simulink model "objectdetectandremember"  (R2023a)
settings: Solver=FixedStepDiscrete  StartTime=0.0  StopTime=200  FixedStep=0.01  RelTol=1e-3
undefined symbols (not defined in the file or in its folder): InputPWM, ticksPerRot, wheelR, WheelSpeed
libraries: mobileRoboticsTrainingLib x7, slpidlib x3
settings Model: Creator=Boitumelo  LastModifiedBy=Nate
settings DebuggingCC: UnconnectedInputMsg=warning  UnconnectedOutputMsg=warning  UnconnectedLineMsg=warning
settings ModelReferenceCC: EnableRefExpFcnMdlSchedulingChecks=on
settings RTWCC: DLArmComputeVersion=19.05

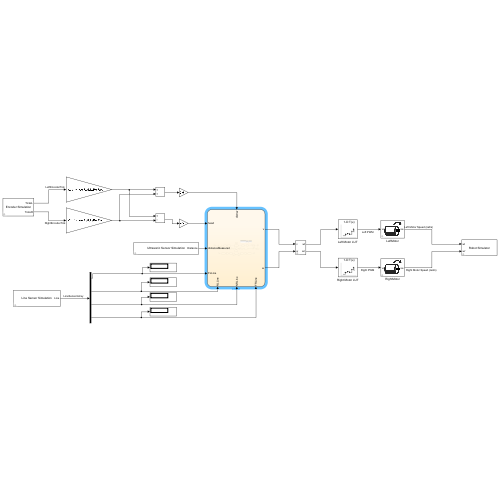
[thumbnail: Simulink's stored preview of the top-level diagram]
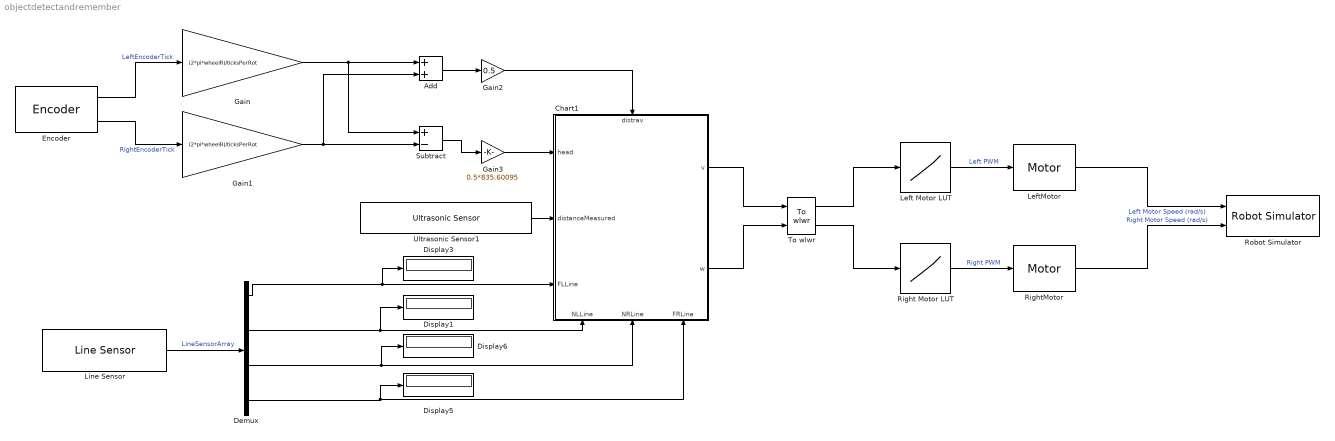
== system objectdetectandremember ==
  Add : Sum
  Chart1 : Stateflow chart  TreatAsAtomicUnit=on
      settings: PortSchema="{\"entries\":[{\"content\":{\"sides\":[{\"content\":{\"connectorIds\":[\"In6\",\"In5\",\"In7\"]},\"type\":\"ConnectorPlacement.EquallySpacedRectSide\",\"uuid\":\"27b5da46-073c-4681-8d78-c3525f10231c\"},{\"content\":{\"connectorIds\":[\"Out1\",\"Out2\"],\"side\":\"RIGHT\"},\"type\":\"ConnectorPlacement.EquallySpacedRectSide\",\"uuid\":\"84cbede5-d577-43ca-a2b5-5c732f2541a7\"},{\"content\":{\"connectorIds\":[\"In4\"],\"side\":\"TOP\"},\"type\":\"ConnectorPlacement.EquallySpacedRectSide\",\"uuid\":\"af8175f1-71d5-4094-87a9-6474fd0e0f31\"},{\"content\":{\"connectorIds\":[\"In1\",\"In2\",\"In3\"],\"side\":\"BOTTOM\"},\"type\":\"ConnectorPlacement.EquallySpacedRectSide\",\"uuid\":\"b4cb3a30-2878-490e-b77d-5d6435204590\"}]},\"type\":\"ConnectorPlacement.EquallySpacedConnector\",\"uuid\":\"b0958b58-2151-4ca2-a50e-e327f459f533\"}],\"packageUris\":[\"http://schema.mathworks.com/mf0/Connector/R2020b\"],\"version\":\"1.0\"}"
  Demux : Demux
  Display{1,3,5..6} (4 alike) : Display
  Encoder : mobileRoboticsTrainingLib/Encoder  axleLength=0.136  wheelR=0.031  ticksPerRot=20
      settings: SourceProductName=Mobile Robotics Training Library
  Gain : Gain  Gain=(2*pi*wheelR)/ticksPerRot
  Gain1 : Gain  Gain=(2*pi*wheelR)/ticksPerRot
  Gain2 : Gain  Gain=0.5
  Gain3 : Gain  Gain=0.5*835.60095
  Left Motor LUT : Lookup_n-D  NumberOfTableDimensions=1  BreakpointsForDimension1=WheelSpeed  Table=InputPWM  InterpMethod=Nearest  ExtrapMethod=Clip  InternalRulePriority=Speed  RndMeth=Simplest
  LeftMotor : mobileRoboticsTrainingLib/Motor  motorPlant=wheelMotorModel  sensorType=Speed
      settings: SourceProductName=Mobile Robotics Training Library
  Line Sensor : mobileRoboticsTrainingLib/Line Sensor  mapVariable=mapForSim  envVal=1000  lineVal=0  sensOff=[0.0643 0.0354; 0.0675 0.005; 0.0675 -0.005; 0.0643 -0.0354]
      settings: SourceProductName=Mobile Robotics Training Library
  Right Motor LUT : Lookup_n-D  NumberOfTableDimensions=1  BreakpointsForDimension1=WheelSpeed  Table=InputPWM  InterpMethod=Nearest  ExtrapMethod=Clip  InternalRulePriority=Speed  RndMeth=Simplest
  RightMotor : mobileRoboticsTrainingLib/Motor  motorPlant=wheelMotorModel  sensorType=Speed
      settings: SourceProductName=Mobile Robotics Training Library
  Robot Simulator : mobileRoboticsTrainingLib/Robot Simulator  Priority=99  mapVar=mapForSim  startX=1  startY=0.2  startTheta=90  axleLength=axleLength  wheelR=wheelR
      link override Wheel Radius: Value=0.031
      link override Wheel Spacing: Value=0.136
  Subtract : Sum  Inputs=+-
  To wlwr : mobileRoboticsTrainingLib/To wlwr  axleLength=axleLength  wheelR=wheelR
      link override change parameters: Gain=[1 +axleLength/2; 1 -axleLength/2]
  Ultrasonic Sensor1 : mobileRoboticsTrainingLib/Ultrasonic Sensor  mapVar=mapForSim  maxSenRange=2  minSenRange=0.02  senRes=0.01  sensOff=[0 0]
      link override Look up Distance Value/Subsystem/Look up Sensor Value/Lookup Obstacle Map/Direct Lookup Table (n-D): DiagnosticForOutOfRangeInput=Warning  TableIsInput=off
      settings: SourceProductName=Mobile Robotics Training Library
  wires:
  Right Motor LUT/1 -> RightMotor/1  "Right PWM"
  Left Motor LUT/1 -> LeftMotor/1  "Left PWM"
  To wlwr/1 -> Left Motor LUT/1
  To wlwr/2 -> Right Motor LUT/1
  RightMotor/1 -> Robot Simulator/2  "Right Motor Speed (rad/s)"
  LeftMotor/1 -> Robot Simulator/1  "Left Motor Speed (rad/s)"
  Line Sensor/1 -> Demux/1  "LineSensorArray"
  Demux/4 -> Display5/1, Chart1/3(FRLine)
  Demux/2 -> Display1/1, Chart1/1(NLLine)
  Demux/3 -> Display6/1, Chart1/2(NRLine)
  Chart1/2(w) -> To wlwr/2
  Chart1/1(v) -> To wlwr/1
  Ultrasonic Sensor1/1 -> Chart1/5(distanceMeasured)
  Gain2/1 -> Chart1/4(distrav)
  Encoder/1 -> Gain/1  "LeftEncoderTick"
  Gain/1 -> Subtract/1, Add/1
  Encoder/2 -> Gain1/1  "RightEncoderTick"
  Add/1 -> Gain2/1
  Demux/1 -> Display3/1, Chart1/7(FLLine)
  Gain1/1 -> Subtract/2, Add/2
  Gain3/1 -> Chart1/6(head)
  Subtract/1 -> Gain3/1

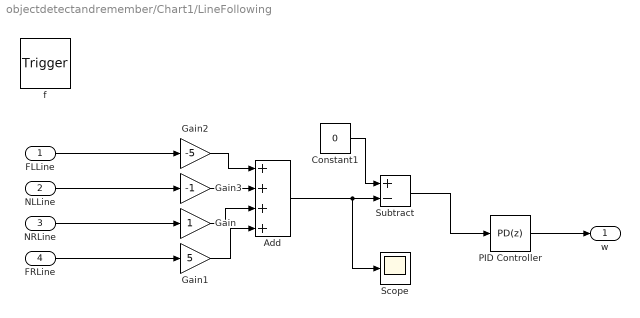
== system objectdetectandremember/Chart1/LineFollowing ==
  FLLine : Inport  OutDataTypeStr=double  PortDimensions=1
  NLLine : Inport  Port=2  OutDataTypeStr=double  PortDimensions=1
  NRLine : Inport  Port=3  OutDataTypeStr=double  PortDimensions=1
  FRLine : Inport  Port=4  OutDataTypeStr=double  PortDimensions=1
  f : TriggerPort  TriggerType=function-call  VariantControl=(inherit)
      settings: CopyFcn=Stateflow.SLINSF.SimulinkMan.removeBlockPreDeleteFcn  PreDeleteFcn=Stateflow.SLINSF.SimulinkMan.unsafePredeleteFcn
  Add : Sum  Inputs=++++
  Constant1 : Constant  Value=0
  Gain : Gain
  Gain1 : Gain  Gain=5
  Gain2 : Gain  Gain=-5
  Gain3 : Gain  Gain=-1
  PID Controller : slpidlib/PID Controller  Controller=PD  Form=Parallel  TimeDomain=Discrete-time  UseExternalTs=off  SampleTime=-1  IntegratorMethod=Forward Euler  FilterMethod=Forward Euler  ControllerParametersSource=internal  P=1  I=0  UseKiTs=off  D=1e-3  N=100  UseFilter=on  TunerSelectOption=Transfer Function Based (PID Tuner App)  InitialConditionSource=internal  InitialConditionForIntegrator=0  InitialConditionForFilter=0  DifferentiatorICPrevScaledInput=0  ExternalReset=none  TrackingMode=off  Kt=1  LimitOutput=off  SatLimitsSource=internal  UpperSaturationLimit=inf  LowerSaturationLimit=-inf  LinearizeAsGain=on  AntiWindupMode=none  Kb=1  LimitIntegrator=off  UpperIntegratorSaturationLimit=inf  LowerIntegratorSaturationLimit=-inf  POutMin=[]  POutMax=[]  IOutMin=[]  IOutMax=[]  DOutMin=[]  DOutMax=[]  NOutMin=[]  NOutMax=[]  SumOutMin=[]  SumOutMax=[]  SaturationOutMin=[]  SaturationOutMax=[]  PParamMin=[]  PParamMax=[]  IParamMin=[]  IParamMax=[]  DParamMin=[]  DParamMax=[]  NParamMin=[]  NParamMax=[]  KbParamMin=[]  KbParamMax=[]  KtParamMin=[]  KtParamMax=[]  KbOutMin=[]  KbOutMax=[]  KtOutMin=[]  KtOutMax=[]  IntegratorOutMin=[]  IntegratorOutMax=[]  FilterOutMin=[]  FilterOutMax=[]  SumI1OutMin=[]  SumI1OutMax=[]  SumI2OutMin=[]  SumI2OutMax=[]  SumI3OutMin=[]  SumI3OutMax=[]  SumI4OutMin=[]  SumI4OutMax=[]  SumDOutMin=[]  SumDOutMax=[]  DifferentiatorOutMin=[]  DifferentiatorOutMax=[]  FilterDiffOutCoefMin=[]  FilterDiffOutCoefMax=[]  ReciprocalOutMin=[]  ReciprocalOutMax=[]  SumDenOutMin=[]  SumDenOutMax=[]  SumNumOutMin=[]  SumNumOutMax=[]  DivideOutMin=[]  DivideOutMax=[]  UdiffTsProdOutMin=[]  UdiffTsProdOutMax=[]  NTsProdOutMin=[]  NTsProdOutMax=[]  UintegralTsProdOutMin=[]  UintegralTsProdOutMax=[]  UngainTsProdOutMin=[]  UngainTsProdOutMax=[]  ClampingZeroOutDataTypeStr=Inherit: Inherit via back propagation  ClampingZeroOutMin=[]  ClampingZeroOutMax=[]  FilterDenConstantOutDataTypeStr=Inherit: Inherit via back propagation  FilterDenConstantOutMin=[]  FilterDenConstantOutMax=[]  PCopyOutDataTypeStr=Inherit: Inherit via back propagation  PCopyOutMin=[]  PCopyOutMax=[]  NCopyOutDataTypeStr=Inherit: Inherit via back propagation  NCopyOutMin=[]  NCopyOutMax=[]  IntegratorContinuousStateAttributes=''  IntegratorStateMustResolveToSignalObject=off  IntegratorRTWStateStorageClass=Auto  FilterContinuousStateAttributes=''  FilterStateMustResolveToSignalObject=off  FilterRTWStateStorageClass=Auto  ParallelPVariant=InternalParameters  IdealPVariant=Disabled  IVariant=Disabled  DVariant=InternalParameters  IntegratorVariant=Disabled  SatVariant=Disabled  AWVariant=Disabled  PCopyVariant=Disabled  TRVariant=Disabled  FdbkBlocksVariant=Forward  IdealPFdbkVariant=Disabled  SatFdbkVariant=Disabled  DerivativeFilterVariant=ForwardEulerFilter  NVariant=InternalParameters  NCopyVariant=Disabled  FilterICVariant=InternalICsFilter  IntegratorICVariant=Disabled  ExternalResetVariant=Disabled  TRSumVariant=Passthrough  SumFdbkVariant=Disabled  SumVariant=Sum_PD  TsampFilterVariant=InternalTs  TsampNgainVariant=Passthrough  TsampIntegralVariant=Disabled_SignalSpec  ExternalSaturationOutDataTypeStr=Inherit: Same as second input
  Scope : Scope
  Subtract : Sum  Inputs=+-
  w : Outport
  wires:
  Gain1/1 -> Add/4
  NRLine/1 -> Gain/1
  Subtract/1 -> PID Controller/1
  Constant1/1 -> Subtract/1
  Gain3/1 -> Add/2
  PID Controller/1 -> w/1
  Gain/1 -> Add/3
  Add/1 -> Scope/1, Subtract/2
  FLLine/1 -> Gain2/1
  Gain2/1 -> Add/1
  FRLine/1 -> Gain1/1
  NLLine/1 -> Gain3/1

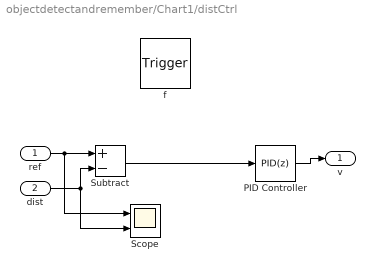
== system objectdetectandremember/Chart1/distCtrl ==
  ref : Inport  OutDataTypeStr=double  PortDimensions=1
  dist : Inport  Port=2  OutDataTypeStr=double  PortDimensions=1
  f : TriggerPort  TriggerType=function-call  VariantControl=(inherit)
      settings: CopyFcn=Stateflow.SLINSF.SimulinkMan.removeBlockPreDeleteFcn  PreDeleteFcn=Stateflow.SLINSF.SimulinkMan.unsafePredeleteFcn
  PID Controller : slpidlib/PID Controller  Controller=PID  Form=Parallel  TimeDomain=Discrete-time  UseExternalTs=off  SampleTime=-1  IntegratorMethod=Forward Euler  FilterMethod=Forward Euler  ControllerParametersSource=internal  P=1.3  I=0.3  UseKiTs=off  D=0.001  N=100  UseFilter=on  TunerSelectOption=Transfer Function Based (PID Tuner App)  InitialConditionSource=internal  InitialConditionForIntegrator=0  InitialConditionForFilter=0  DifferentiatorICPrevScaledInput=0  ExternalReset=none  TrackingMode=off  Kt=1  LimitOutput=on  SatLimitsSource=internal  UpperSaturationLimit=0.32  LowerSaturationLimit=-0.32  LinearizeAsGain=on  AntiWindupMode=clamping  Kb=1  LimitIntegrator=off  UpperIntegratorSaturationLimit=inf  LowerIntegratorSaturationLimit=-inf  POutMin=[]  POutMax=[]  IOutMin=[]  IOutMax=[]  DOutMin=[]  DOutMax=[]  NOutMin=[]  NOutMax=[]  SumOutMin=[]  SumOutMax=[]  SaturationOutMin=[]  SaturationOutMax=[]  PParamMin=[]  PParamMax=[]  IParamMin=[]  IParamMax=[]  DParamMin=[]  DParamMax=[]  NParamMin=[]  NParamMax=[]  KbParamMin=[]  KbParamMax=[]  KtParamMin=[]  KtParamMax=[]  KbOutMin=[]  KbOutMax=[]  KtOutMin=[]  KtOutMax=[]  IntegratorOutMin=[]  IntegratorOutMax=[]  FilterOutMin=[]  FilterOutMax=[]  SumI1OutMin=[]  SumI1OutMax=[]  SumI2OutMin=[]  SumI2OutMax=[]  SumI3OutMin=[]  SumI3OutMax=[]  SumI4OutMin=[]  SumI4OutMax=[]  SumDOutMin=[]  SumDOutMax=[]  DifferentiatorOutMin=[]  DifferentiatorOutMax=[]  FilterDiffOutCoefMin=[]  FilterDiffOutCoefMax=[]  ReciprocalOutMin=[]  ReciprocalOutMax=[]  SumDenOutMin=[]  SumDenOutMax=[]  SumNumOutMin=[]  SumNumOutMax=[]  DivideOutMin=[]  DivideOutMax=[]  UdiffTsProdOutMin=[]  UdiffTsProdOutMax=[]  NTsProdOutMin=[]  NTsProdOutMax=[]  UintegralTsProdOutMin=[]  UintegralTsProdOutMax=[]  UngainTsProdOutMin=[]  UngainTsProdOutMax=[]  ClampingZeroOutDataTypeStr=Inherit: Inherit via back propagation  ClampingZeroOutMin=[]  ClampingZeroOutMax=[]  FilterDenConstantOutDataTypeStr=Inherit: Inherit via back propagation  FilterDenConstantOutMin=[]  FilterDenConstantOutMax=[]  PCopyOutDataTypeStr=Inherit: Inherit via back propagation  PCopyOutMin=[]  PCopyOutMax=[]  NCopyOutDataTypeStr=Inherit: Inherit via back propagation  NCopyOutMin=[]  NCopyOutMax=[]  IntegratorContinuousStateAttributes=''  IntegratorStateMustResolveToSignalObject=off  IntegratorRTWStateStorageClass=Auto  FilterContinuousStateAttributes=''  FilterStateMustResolveToSignalObject=off  FilterRTWStateStorageClass=Auto  ParallelPVariant=InternalParameters  IdealPVariant=Disabled  IVariant=InternalParameters  DVariant=InternalParameters  IntegratorVariant=Discrete  SatVariant=Enabled  AWVariant=DiscClampingParallel  PCopyVariant=Disabled  TRVariant=Disabled  FdbkBlocksVariant=Forward  IdealPFdbkVariant=Disabled  SatFdbkVariant=Disabled  DerivativeFilterVariant=ForwardEulerFilter  NVariant=InternalParameters  NCopyVariant=Disabled  FilterICVariant=InternalICsFilter  IntegratorICVariant=InternalICs  ExternalResetVariant=Disabled  TRSumVariant=Passthrough  SumFdbkVariant=Disabled  SumVariant=Sum_PID  TsampFilterVariant=InternalTs  TsampNgainVariant=Passthrough  TsampIntegralVariant=Disabled_SignalSpec  ExternalSaturationOutDataTypeStr=Inherit: Same as second input
  Scope : Scope  NumInputPorts=2
  Subtract : Sum  Inputs=+-
  v : Outport
  wires:
  ref/1 -> Scope/1, Subtract/1
  dist/1 -> Scope/2, Subtract/2
  PID Controller/1 -> v/1
  Subtract/1 -> PID Controller/1

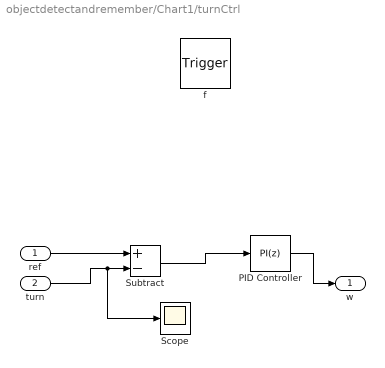
== system objectdetectandremember/Chart1/turnCtrl ==
  ref : Inport  OutDataTypeStr=double  PortDimensions=1
  turn : Inport  Port=2  OutDataTypeStr=double  PortDimensions=1
  f : TriggerPort  TriggerType=function-call  VariantControl=(inherit)
      settings: CopyFcn=Stateflow.SLINSF.SimulinkMan.removeBlockPreDeleteFcn  PreDeleteFcn=Stateflow.SLINSF.SimulinkMan.unsafePredeleteFcn
  PID Controller : slpidlib/PID Controller  Controller=PI  Form=Parallel  TimeDomain=Discrete-time  UseExternalTs=off  SampleTime=-1  IntegratorMethod=Forward Euler  FilterMethod=Forward Euler  ControllerParametersSource=internal  P=0.1  I=0.0001  UseKiTs=off  D=0  N=100  UseFilter=on  TunerSelectOption=Transfer Function Based (PID Tuner App)  InitialConditionSource=internal  InitialConditionForIntegrator=0  InitialConditionForFilter=0  DifferentiatorICPrevScaledInput=0  ExternalReset=none  TrackingMode=off  Kt=1  LimitOutput=on  SatLimitsSource=internal  UpperSaturationLimit=0.32  LowerSaturationLimit=-0.32  LinearizeAsGain=on  AntiWindupMode=clamping  Kb=1  LimitIntegrator=off  UpperIntegratorSaturationLimit=inf  LowerIntegratorSaturationLimit=-inf  POutMin=[]  POutMax=[]  IOutMin=[]  IOutMax=[]  DOutMin=[]  DOutMax=[]  NOutMin=[]  NOutMax=[]  SumOutMin=[]  SumOutMax=[]  SaturationOutMin=[]  SaturationOutMax=[]  PParamMin=[]  PParamMax=[]  IParamMin=[]  IParamMax=[]  DParamMin=[]  DParamMax=[]  NParamMin=[]  NParamMax=[]  KbParamMin=[]  KbParamMax=[]  KtParamMin=[]  KtParamMax=[]  KbOutMin=[]  KbOutMax=[]  KtOutMin=[]  KtOutMax=[]  IntegratorOutMin=[]  IntegratorOutMax=[]  FilterOutMin=[]  FilterOutMax=[]  SumI1OutMin=[]  SumI1OutMax=[]  SumI2OutMin=[]  SumI2OutMax=[]  SumI3OutMin=[]  SumI3OutMax=[]  SumI4OutMin=[]  SumI4OutMax=[]  SumDOutMin=[]  SumDOutMax=[]  DifferentiatorOutMin=[]  DifferentiatorOutMax=[]  FilterDiffOutCoefMin=[]  FilterDiffOutCoefMax=[]  ReciprocalOutMin=[]  ReciprocalOutMax=[]  SumDenOutMin=[]  SumDenOutMax=[]  SumNumOutMin=[]  SumNumOutMax=[]  DivideOutMin=[]  DivideOutMax=[]  UdiffTsProdOutMin=[]  UdiffTsProdOutMax=[]  NTsProdOutMin=[]  NTsProdOutMax=[]  UintegralTsProdOutMin=[]  UintegralTsProdOutMax=[]  UngainTsProdOutMin=[]  UngainTsProdOutMax=[]  ClampingZeroOutDataTypeStr=Inherit: Inherit via back propagation  ClampingZeroOutMin=[]  ClampingZeroOutMax=[]  FilterDenConstantOutDataTypeStr=Inherit: Inherit via back propagation  FilterDenConstantOutMin=[]  FilterDenConstantOutMax=[]  PCopyOutDataTypeStr=Inherit: Inherit via back propagation  PCopyOutMin=[]  PCopyOutMax=[]  NCopyOutDataTypeStr=Inherit: Inherit via back propagation  NCopyOutMin=[]  NCopyOutMax=[]  IntegratorContinuousStateAttributes=''  IntegratorStateMustResolveToSignalObject=off  IntegratorRTWStateStorageClass=Auto  FilterContinuousStateAttributes=''  FilterStateMustResolveToSignalObject=off  FilterRTWStateStorageClass=Auto  ParallelPVariant=InternalParameters  IdealPVariant=Disabled  IVariant=InternalParameters  DVariant=Disabled  IntegratorVariant=Discrete  SatVariant=Enabled  AWVariant=DiscClampingParallel  PCopyVariant=Disabled  TRVariant=Disabled  FdbkBlocksVariant=Forward  IdealPFdbkVariant=Disabled  SatFdbkVariant=Disabled  DerivativeFilterVariant=Disabled  NVariant=Disabled  NCopyVariant=Disabled_SignalSpec  FilterICVariant=Disabled  IntegratorICVariant=InternalICs  ExternalResetVariant=Disabled  TRSumVariant=Passthrough  SumFdbkVariant=Disabled  SumVariant=Sum_PI  TsampFilterVariant=InternalTs  TsampNgainVariant=Passthrough  TsampIntegralVariant=Disabled_SignalSpec  ExternalSaturationOutDataTypeStr=Inherit: Same as second input
  Scope : Scope
  Subtract : Sum  Inputs=+-
  w : Outport
  wires:
  turn/1 -> Scope/1, Subtract/2
  Subtract/1 -> PID Controller/1
  ref/1 -> Subtract/1
  PID Controller/1 -> w/1

== stateflow chart objectdetectandremember/Chart1 ==
  state w = LineFollowing(FLLine, NLLine, NRLine, FRLine) [function]
  state w = turnCtrl(ref,turn) [function]
  state v = distCtrl(ref,dist) [function]
  state Variables
    entry:
    current=1
    iDist = distrav
    turn=0
  state TurnR
    entry:
    v=0
    turn=turn+1
    iHead=head
    during:
    w=turnCtrl(90, head - iHead)
  state MoveL1
    entry:
    v=0.3
    during:
    w =LineFollowing(FLLine, NLLine, NRLine, FRLine)
  state TurnL
    entry:
    v=0
    turn=turn+1
    iHead=head
    during:
    w=turnCtrl(-90, head - iHead)
  state MoveR1
    entry:
    v=0.3
    during:
    w =LineFollowing(FLLine, NLLine, NRLine, FRLine)
  state LeftIntersect
    entry:
    iDist=distrav
    w=0
    during:
    v=distCtrl(iDist+0.0643,distrav)
  state Start
    entry:
    v=0.3
    during:
    w =LineFollowing(FLLine, NLLine, NRLine, FRLine)
  state DetectlineR
    entry:
    v=0
    w=0
  state RightIntersect
    entry:
    iDist=distrav
    w=0
    during:
    v=distCtrl(iDist+0.0643,distrav)
  state DetectlineL
    entry:
    v=0
    w=0
  state deadendR1
    entry:
    v=0
    w=0
    current=current+1
  state deadendR
    entry:
    v=0
    w=0
    current = current+1
  state Detectline
    entry:
    v=0
    w=0
  state MoveR2
    entry:
    v=0.3
    during:
    w =LineFollowing(FLLine, NLLine, NRLine, FRLine)
  state MoveL2
    entry:
    v=0.3
    during:
    w =LineFollowing(FLLine, NLLine, NRLine, FRLine)
  state TurnR1
    entry:
    v=0
    iHead=head
    during:
    w=turnCtrl(90, head - iHead)
  state TurnL1
    entry:
    v=0
    iHead=head
    during:
    w=turnCtrl(-90, head - iHead)
  state RightIntersect1
    entry:
    iDist=distrav
    w=0
    during:
    v=distCtrl(iDist+0.0643,distrav)
  state LeftIntersect1
    entry:
    iDist=distrav
    w=0
    during:
    v=distCtrl(iDist+0.0643,distrav)
  state savedistobjectR
    entry:
    objectdist(current)=distanceMeasured
    current=current + 1
  state savedistobjectL
    entry:
    objectdist(current)=distanceMeasured
    current=current + 1
  state UturnR
    entry:
    iHead=head
    during:
    w=turnCtrl(180, head - iHead)
  state UturnL
    entry:
    iHead=head
    during:
    w=turnCtrl(180, head - iHead)
  state InitialmoveR
    entry:
    v=0.3
  state InitialmoveL
    entry:
    v=0.3
  state Uturnend
    entry:
    iHead=head
    during:
    w=turnCtrl(180, head - iHead)
    short = min(objectdist)
    Sturn = find(objectdist==short)
    ignore = 1+turn-Sturn(1)
  state MoveL3
    entry:
    v=0.3
    during:
    w =LineFollowing(FLLine, NLLine, NRLine, FRLine)
  state MoveRFinal
    entry:
    v=0.3
    during:
    w =LineFollowing(FLLine, NLLine, NRLine, FRLine)
  state MoveFinal
    entry:
    v=0.3
    during:
    w =LineFollowing(FLLine, NLLine, NRLine, FRLine)
  state TurnL2
    entry:
    v=0
    turn=turn+1
    iHead=head
    during:
    w=turnCtrl(-90, head - iHead)
  state TurnRFinal
    entry:
    v=0
    turn=turn+1
    iHead=head
    during:
    w=turnCtrl(90, head - iHead)
  state LeftIntersectFinal
    entry:
    iDist=distrav
    w=0
    ignore = ignore-1
    during:
    v=distCtrl(iDist+0.0643,distrav)
  state RightIntersectFinal
    entry:
    iDist=distrav
    w=0
    ignore = ignore-1
    during:
    v=distCtrl(iDist+0.0643,distrav)
  state DetectlineLFinal
    entry:
    v=0
    w=0
  state DetectlineRFinal
    entry:
    v=0
    w=0
  state PastTurnL
    v=0.24
  state PastTurnR
    v=0.24
  (default) -> Variables
  Variables -> Start
  TurnR -> MoveR1 : [after(2,sec)]
  MoveR1 -> DetectlineR [order 2] : [FRLine==0 && FLLine==0]
  Start -> LeftIntersect [order 3] : [after(0.6,sec)&&FLLine==0 && FRLine~=0]
  TurnL -> MoveL1 : [after(2,sec)]
  MoveL1 -> DetectlineL [order 1] : [FRLine==0 && FLLine==0]
  Start -> RightIntersect [order 1] : [after(0.6,sec)&&FRLine==0 && FLLine~=0]
  LeftIntersect -> TurnL [order 1] : [after(1.5,sec)]
  RightIntersect -> TurnR [order 1] : [after(3,sec)]
  DetectlineR -> savedistobjectR : [after(4,sec)]
  MoveR1 -> deadendR [order 1] : [after(0.5,sec) &&FRLine==1000&&FLLine==1000&&NLLine==1000&&NRLine==1000]
  DetectlineL -> savedistobjectL : [after(4,sec)]
  LeftIntersect -> Detectline [order 2] : [FLLine==0&&FRLine==0]
  MoveL1 -> deadendR1 [order 2] : [after(0.5,sec) &&FRLine==1000&&FLLine==1000&&NLLine==1000&&NRLine==1000]
  RightIntersect -> Detectline [order 2] : [FLLine==0&&FRLine==0]
  InitialmoveL -> Start : [after(0.5,sec)]
  Start -> Detectline [order 2] : [FRLine==0 && FLLine==0]
  InitialmoveR -> Start : [after(0.5,sec)]
  deadendR1 -> UturnL : [after(3,sec)]
  deadendR -> UturnR : [after(3,sec)]
  RightIntersect1 -> TurnR1 : [after(1.5,sec)]
  MoveR2 -> RightIntersect1 : [FRLine==0]
  TurnR1 -> InitialmoveR : [after(4,sec)]
  savedistobjectL -> UturnL : [after(1,sec)]
  UturnR -> MoveR2 : [after(3,sec)]
  savedistobjectR -> UturnR : [after(1,sec)]
  UturnL -> MoveL2 : [after(3,sec)]
  TurnL1 -> InitialmoveL : [after(4,sec)]
  MoveL2 -> LeftIntersect1 : [FLLine==0]
  LeftIntersect1 -> TurnL1 : [after(3,sec)]
  Detectline -> Uturnend : [after(2,sec)]
  Uturnend -> MoveFinal : [after(2,sec)]
  TurnRFinal -> MoveRFinal : [after(2,sec)]
  MoveRFinal -> DetectlineRFinal : [FRLine==0 && FLLine==0]
  RightIntersectFinal -> TurnRFinal [order 2] : [after(1.5,sec)]
  TurnL2 -> MoveL3 : [after(2,sec)]
  MoveFinal -> RightIntersectFinal [order 1] : [FRLine==0 && FLLine~=0]
  MoveFinal -> LeftIntersectFinal [order 2] : [FLLine==0 && FRLine~=0]
  MoveL3 -> DetectlineLFinal : [FRLine==0 && FLLine==0]
  LeftIntersectFinal -> TurnL2 [order 1] : [after(1.5,sec)]
  LeftIntersectFinal -> PastTurnL [order 2] : [ignore~=0]
  RightIntersectFinal -> PastTurnR [order 1] : [ignore~=0]
  PastTurnL -> MoveFinal : [after(0.1,sec)]
  PastTurnR -> MoveFinal : [after(0.1,sec)]
  data: FLLine function_input double size=1; NLLine function_input double size=1; NRLine function_input double size=1; FRLine function_input double size=1; w function_output; ref function_input double size=1; turn function_input double size=1; w function_output; ref function_input double size=1; dist function_input double size=1; v function_output; NLLine input; NRLine input; FRLine input; v output; w output; distrav input; distanceMeasured input; head input; FLLine input; iDist local; iHead local; objectdist local size=1,5 =[3 3 3 3 3]; current local; turn local; Sturn local size=5 [1..5]; ignore local size=5 [1..5]; short local size=5
